simulink model "full_correlator"  (R2022a)
settings: Solver=VariableStepDiscrete  StartTime=0.0  StopTime=4000  RelTol=1e-3
libraries: hdlBasic x2638, hdlSSR x215, hdlDSPIP x4, xbsIndex_r4 x1, xps_library x1
(part 9 of 43)

== system full_correlator/Subsystem2/shared_bram3/sim_mem ==
  addr : Inport
  data : Inport  Port=2
  we : Inport  Port=3
  Data Type Conversion : DataTypeConversion  OutDataTypeStr=single  SaturateOnIntegerOverflow=off  RndMeth=Floor
  Data Type Conversion1 : DataTypeConversion  OutDataTypeStr=double  SaturateOnIntegerOverflow=off  RndMeth=Floor
  Data Type Conversion2 : DataTypeConversion  OutDataTypeStr=boolean  SaturateOnIntegerOverflow=off  RndMeth=Floor
  sfunc : M-S-Function  FunctionName=shared_bram_sim_sfunc  Parameters=depth_bits, latency, init_vals  mask{depth_bits=addr_width, latency=csp_latency, init_vals=init_vals}
      mask prompts: depth_bits "Depth (2^?):"; latency "Latency (>=1):"; init_vals "Initial values:"
      mask Callback latency:
      | latency = str2double(get_param(gcb, 'latency'));
      | if latency < 1
      |     errordlg('Cannot have latency less than one.');
      |     set_param(gcb, 'latency', '1');
      | end
  sim_addr : hdlBasic/Gateway Out  inherit_from_input=off  hdl_port=off  rows=1  columns=1  UseAsDAC=off  DACChannel='1'  interface=None  automatic_assignment=on  address_offset=hex2dec('00')  intf_name=''  intf_description=''  timing_constraint=None  locs_specified=off  LOCs={}  io_standard={}  XmcBlockStatus=1  maskContainerNames=group4  block_type=gatewayout  block_config=sysgen:gateway_out_config  block_width_w=590  block_height_w=620  block_width=620  block_height=750
  sim_data : hdlBasic/Gateway Out  inherit_from_input=off  hdl_port=off  rows=1  columns=1  UseAsDAC=off  DACChannel='1'  interface=None  automatic_assignment=on  address_offset=hex2dec('00')  intf_name=''  intf_description=''  timing_constraint=None  locs_specified=off  LOCs={}  io_standard={}  XmcBlockStatus=1  maskContainerNames=group4  block_type=gatewayout  block_config=sysgen:gateway_out_config  block_width_w=590  block_height_w=620  block_width=620  block_height=750
  sim_we : hdlBasic/Gateway Out  inherit_from_input=off  hdl_port=off  rows=1  columns=1  UseAsDAC=off  DACChannel='1'  interface=None  automatic_assignment=on  address_offset=hex2dec('00')  intf_name=''  intf_description=''  timing_constraint=None  locs_specified=off  LOCs={}  io_standard={}  XmcBlockStatus=1  maskContainerNames=group4  block_type=gatewayout  block_config=sysgen:gateway_out_config  block_width_w=590  block_height_w=620  block_width=620  block_height=750
  data_out : Outport  VectorParamsAs1DForOutWhenUnconnected=off
  wires:
  sfunc/1 -> data_out/1  "output"
  Data Type Conversion2/1 -> sfunc/3  "we"
  Data Type Conversion1/1 -> sfunc/2  "data_in"
  Data Type Conversion/1 -> sfunc/1  "addr"
  sim_we/1 -> Data Type Conversion2/1
  sim_data/1 -> Data Type Conversion1/1
  sim_addr/1 -> Data Type Conversion/1
  we/1 -> sim_we/1
  data/1 -> sim_data/1
  addr/1 -> sim_addr/1

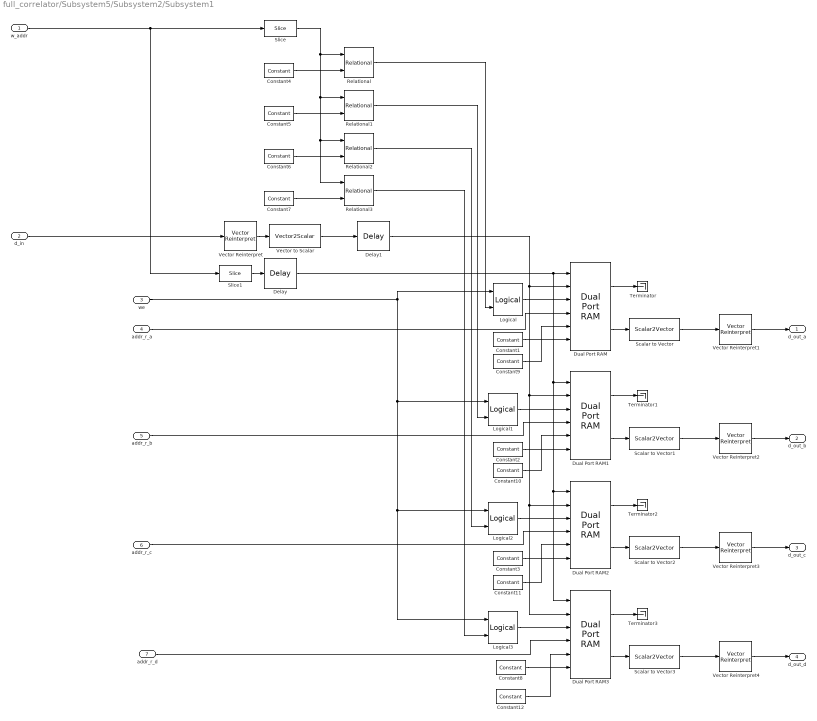
== system full_correlator/Subsystem5/Subsystem2/Subsystem1 ==
  w_addr : Inport
  d_in : Inport  Port=2
  we : Inport  Port=3
  addr_r_a : Inport  Port=4
  addr_r_b : Inport  Port=5
  addr_r_c : Inport  Port=6
  addr_r_d : Inport  Port=7
  Constant{1..3,8} (4 alike) : hdlBasic/Constant  const=0  gui_display_data_type=Boolean  arith_type=Boolean  n_bits=16  bin_pt=14  preci_type=Single  exp_width=8  frac_width=24  explicit_period=on  period=1  XmcBlockStatus=1  maskContainerNames=tabcontainer1  block_type=constant  block_config=sysgen:Constant_config
  Constant{9..12} (4 alike) : hdlBasic/Constant  const=0  gui_display_data_type=Fixed-point  arith_type=Unsigned  n_bits=288  bin_pt=0  preci_type=Single  exp_width=8  frac_width=24  explicit_period=on  period=1  XmcBlockStatus=1  maskContainerNames=tabcontainer1  block_type=constant  block_config=sysgen:Constant_config
  Constant4 : hdlBasic/Constant  const=0  gui_display_data_type=Fixed-point  arith_type=Unsigned  n_bits=2  bin_pt=0  preci_type=Single  exp_width=8  frac_width=24  explicit_period=on  period=1  XmcBlockStatus=1  maskContainerNames=tabcontainer1  block_type=constant  block_config=sysgen:Constant_config
  Constant5 : hdlBasic/Constant  const=1  gui_display_data_type=Fixed-point  arith_type=Unsigned  n_bits=2  bin_pt=0  preci_type=Single  exp_width=8  frac_width=24  explicit_period=on  period=1  XmcBlockStatus=1  maskContainerNames=tabcontainer1  block_type=constant  block_config=sysgen:Constant_config
  Constant6 : hdlBasic/Constant  const=2  gui_display_data_type=Fixed-point  arith_type=Unsigned  n_bits=2  bin_pt=0  preci_type=Single  exp_width=8  frac_width=24  explicit_period=on  period=1  XmcBlockStatus=1  maskContainerNames=tabcontainer1  block_type=constant  block_config=sysgen:Constant_config
  Constant7 : hdlBasic/Constant  const=3  gui_display_data_type=Fixed-point  arith_type=Unsigned  n_bits=2  bin_pt=0  preci_type=Single  exp_width=8  frac_width=24  explicit_period=on  period=1  XmcBlockStatus=1  maskContainerNames=tabcontainer1  block_type=constant  block_config=sysgen:Constant_config
  Delay : hdlBasic/Delay  rst=off  en=off  latency=2  reg_retiming=off  XmcBlockStatus=1  maskContainerNames=group1  block_type=delay  block_config=sysgen:Delay_config
  Delay1 : hdlBasic/Delay  rst=off  en=off  latency=2  reg_retiming=off  XmcBlockStatus=1  maskContainerNames=group1  block_type=delay  block_config=sysgen:Delay_config
  Dual Port RAM{,1..3} (4 alike) : hdlBasic/Dual Port RAM  depth=16  initVector=zeros(1, 16)  distributed_mem=Block RAM  init_a=0  init_b=0  rst_a=off  rst_b=off  en_a=off  en_b=off  latency=1  write_mode_A=Read After Write  write_mode_B=Read After Write  explicit_period=[]  period=[]  simulation_type=fast_sim  XmcBlockStatus=1  maskContainerNames=tabcontainer1  block_type=dpram  block_config=sysgen:Dpram_config  optimize=Area
      settings: infoedit=[]
  Logical{,1..3} (4 alike) : hdlBasic/Logical  logical_function=AND  inputs=2  en=off  latency=1  precision=Full  arith_type=Unsigned  n_bits=16  bin_pt=0  align_bp=on  overflow=[]  quantization=[]  XmcBlockStatus=1  maskContainerNames=tabcontainer1  block_type=logical  block_config=sysgen:Logical_config
  Relational{,1..3} (4 alike) : hdlBasic/Relational  mode=a=b  op_type=Bool  en=off  latency=1  XmcBlockStatus=1  maskContainerNames=tabcontainer1  block_type=relational  block_config=sysgen:Relational_config
  Scalar to Vector{,1..3} (4 alike) : hdlSSR/Scalar2Vector  Width=18  sg_ssr=16  block_type=scalar2vector_ssr  XmcBlockStatus=1  sg_ssr_prev=16  maskContainerNames=group1
  Slice : hdlBasic/Slice  nbits=2  boolean_output=off  mode=Upper Bit Location + Width  bit1=0  base1=MSB of Input  bit0=0  base0=LSB of Input  XmcBlockStatus=1  maskContainerNames=group1  block_type=slice  block_config=sysgen:Slice_config
  Slice1 : hdlBasic/Slice  nbits=4  boolean_output=off  mode=Upper Bit Location + Width  bit1=-2  base1=MSB of Input  bit0=0  base0=LSB of Input  XmcBlockStatus=1  maskContainerNames=group1  block_type=slice  block_config=sysgen:Slice_config
  Terminator{,1..3} (4 alike) : Terminator
  Vector Reinterpret : hdlSSR/Vector Reinterpret  force_arith_type=on  arith_type=Unsigned  force_bin_pt=on  bin_pt=0  sg_ssr=16  block_type=reinterpret_ssr  XmcBlockStatus=1  sg_ssr_prev=16  maskContainerNames=group1
  Vector Reinterpret{1..4} (4 alike) : hdlSSR/Vector Reinterpret  force_arith_type=on  arith_type="Signed  (2's comp)"  force_bin_pt=on  bin_pt=17  sg_ssr=16  block_type=reinterpret_ssr  XmcBlockStatus=1  sg_ssr_prev=16  maskContainerNames=group1
  Vector to Scalar : hdlSSR/Vector2Scalar  sg_ssr=16  block_type=vector2scalar_ssr  XmcBlockStatus=1  sg_ssr_prev=16  maskContainerNames=group1
  d_out_a : Outport
  d_out_b : Outport  Port=2
  d_out_c : Outport  Port=3
  d_out_d : Outport  Port=4
  wires:
  addr_r_b/1 -> Dual Port RAM1/4
  Constant12/1 -> Dual Port RAM3/5
  addr_r_c/1 -> Dual Port RAM2/4
  Relational/1 -> Logical/2
  Constant6/1 -> Relational2/2
  Dual Port RAM1/1 -> Terminator1/1
  Constant11/1 -> Dual Port RAM2/5
  Vector Reinterpret/1 -> Vector to Scalar/1
  Relational3/1 -> Logical3/2
  Constant7/1 -> Relational3/2
  Dual Port RAM/1 -> Terminator/1
  Delay/1 -> Dual Port RAM3/1, Dual Port RAM2/1, Dual Port RAM1/1, Dual Port RAM/1
  Vector to Scalar/1 -> Delay1/1
  Logical2/1 -> Dual Port RAM2/3
  d_in/1 -> Vector Reinterpret/1
  Constant3/1 -> Dual Port RAM2/6
  Dual Port RAM1/2 -> Scalar to Vector1/1
  Delay1/1 -> Dual Port RAM3/2, Dual Port RAM2/2, Dual Port RAM1/2, Dual Port RAM/2
  Relational1/1 -> Logical1/2
  we/1 -> Logical3/1, Logical2/1, Logical1/1, Logical/1
  Slice/1 -> Relational3/1, Relational2/1, Relational1/1, Relational/1
  Constant9/1 -> Dual Port RAM/5
  Constant1/1 -> Dual Port RAM/6
  Dual Port RAM2/1 -> Terminator2/1
  Constant10/1 -> Dual Port RAM1/5
  w_addr/1 -> Slice1/1, Slice/1
  Dual Port RAM3/2 -> Scalar to Vector3/1
  Logical/1 -> Dual Port RAM/3
  Constant2/1 -> Dual Port RAM1/6
  Constant8/1 -> Dual Port RAM3/6
  Constant4/1 -> Relational/2
  Dual Port RAM3/1 -> Terminator3/1
  Logical1/1 -> Dual Port RAM1/3
  Logical3/1 -> Dual Port RAM3/3
  Constant5/1 -> Relational1/2
  Dual Port RAM2/2 -> Scalar to Vector2/1
  addr_r_d/1 -> Dual Port RAM3/4
  Slice1/1 -> Delay/1
  Relational2/1 -> Logical2/2
  addr_r_a/1 -> Dual Port RAM/4
  Dual Port RAM/2 -> Scalar to Vector/1
  Scalar to Vector/1 -> Vector Reinterpret1/1
  Scalar to Vector1/1 -> Vector Reinterpret2/1
  Scalar to Vector2/1 -> Vector Reinterpret3/1
  Scalar to Vector3/1 -> Vector Reinterpret4/1
  Vector Reinterpret1/1 -> d_out_a/1
  Vector Reinterpret2/1 -> d_out_b/1
  Vector Reinterpret3/1 -> d_out_c/1
  Vector Reinterpret4/1 -> d_out_d/1

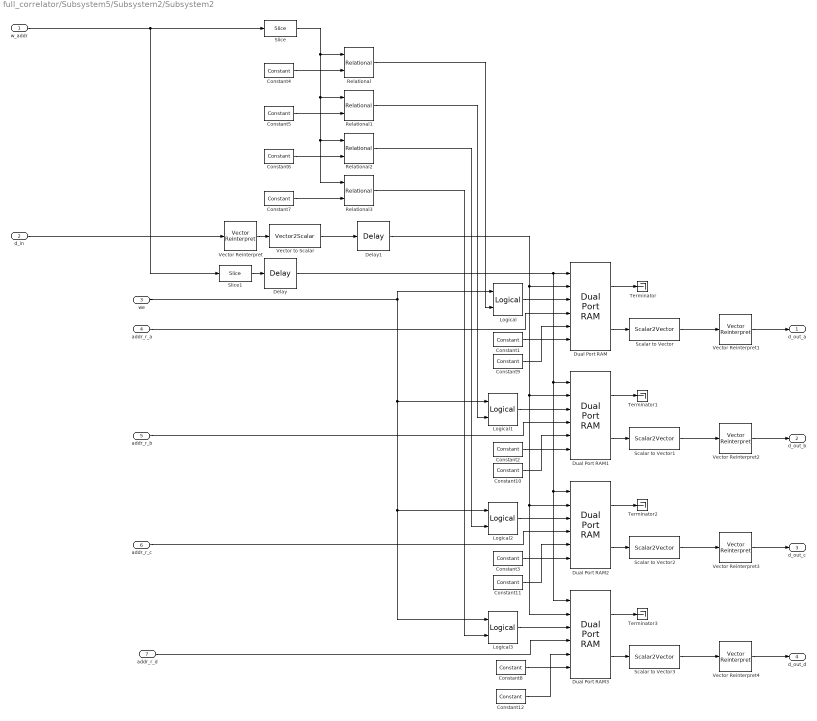
== system full_correlator/Subsystem5/Subsystem2/Subsystem2 ==
  w_addr : Inport
  d_in : Inport  Port=2
  we : Inport  Port=3
  addr_r_a : Inport  Port=4
  addr_r_b : Inport  Port=5
  addr_r_c : Inport  Port=6
  addr_r_d : Inport  Port=7
  Constant{1..3,8} (4 alike) : hdlBasic/Constant  const=0  gui_display_data_type=Boolean  arith_type=Boolean  n_bits=16  bin_pt=14  preci_type=Single  exp_width=8  frac_width=24  explicit_period=on  period=1  XmcBlockStatus=1  maskContainerNames=tabcontainer1  block_type=constant  block_config=sysgen:Constant_config
  Constant{9..12} (4 alike) : hdlBasic/Constant  const=0  gui_display_data_type=Fixed-point  arith_type=Unsigned  n_bits=288  bin_pt=0  preci_type=Single  exp_width=8  frac_width=24  explicit_period=on  period=1  XmcBlockStatus=1  maskContainerNames=tabcontainer1  block_type=constant  block_config=sysgen:Constant_config
  Constant4 : hdlBasic/Constant  const=0  gui_display_data_type=Fixed-point  arith_type=Unsigned  n_bits=2  bin_pt=0  preci_type=Single  exp_width=8  frac_width=24  explicit_period=on  period=1  XmcBlockStatus=1  maskContainerNames=tabcontainer1  block_type=constant  block_config=sysgen:Constant_config
  Constant5 : hdlBasic/Constant  const=1  gui_display_data_type=Fixed-point  arith_type=Unsigned  n_bits=2  bin_pt=0  preci_type=Single  exp_width=8  frac_width=24  explicit_period=on  period=1  XmcBlockStatus=1  maskContainerNames=tabcontainer1  block_type=constant  block_config=sysgen:Constant_config
  Constant6 : hdlBasic/Constant  const=2  gui_display_data_type=Fixed-point  arith_type=Unsigned  n_bits=2  bin_pt=0  preci_type=Single  exp_width=8  frac_width=24  explicit_period=on  period=1  XmcBlockStatus=1  maskContainerNames=tabcontainer1  block_type=constant  block_config=sysgen:Constant_config
  Constant7 : hdlBasic/Constant  const=3  gui_display_data_type=Fixed-point  arith_type=Unsigned  n_bits=2  bin_pt=0  preci_type=Single  exp_width=8  frac_width=24  explicit_period=on  period=1  XmcBlockStatus=1  maskContainerNames=tabcontainer1  block_type=constant  block_config=sysgen:Constant_config
  Delay : hdlBasic/Delay  rst=off  en=off  latency=2  reg_retiming=off  XmcBlockStatus=1  maskContainerNames=group1  block_type=delay  block_config=sysgen:Delay_config
  Delay1 : hdlBasic/Delay  rst=off  en=off  latency=2  reg_retiming=off  XmcBlockStatus=1  maskContainerNames=group1  block_type=delay  block_config=sysgen:Delay_config
  Dual Port RAM{,1..3} (4 alike) : hdlBasic/Dual Port RAM  depth=16  initVector=zeros(1, 16)  distributed_mem=Block RAM  init_a=0  init_b=0  rst_a=off  rst_b=off  en_a=off  en_b=off  latency=1  write_mode_A=Read After Write  write_mode_B=Read After Write  explicit_period=[]  period=[]  simulation_type=fast_sim  XmcBlockStatus=1  maskContainerNames=tabcontainer1  block_type=dpram  block_config=sysgen:Dpram_config  optimize=Area
      settings: infoedit=[]
  Logical{,1..3} (4 alike) : hdlBasic/Logical  logical_function=AND  inputs=2  en=off  latency=1  precision=Full  arith_type=Unsigned  n_bits=16  bin_pt=0  align_bp=on  overflow=[]  quantization=[]  XmcBlockStatus=1  maskContainerNames=tabcontainer1  block_type=logical  block_config=sysgen:Logical_config
  Relational{,1..3} (4 alike) : hdlBasic/Relational  mode=a=b  op_type=Bool  en=off  latency=1  XmcBlockStatus=1  maskContainerNames=tabcontainer1  block_type=relational  block_config=sysgen:Relational_config
  Scalar to Vector{,1..3} (4 alike) : hdlSSR/Scalar2Vector  Width=18  sg_ssr=16  block_type=scalar2vector_ssr  XmcBlockStatus=1  sg_ssr_prev=16  maskContainerNames=group1
  Slice : hdlBasic/Slice  nbits=2  boolean_output=off  mode=Upper Bit Location + Width  bit1=0  base1=MSB of Input  bit0=0  base0=LSB of Input  XmcBlockStatus=1  maskContainerNames=group1  block_type=slice  block_config=sysgen:Slice_config
  Slice1 : hdlBasic/Slice  nbits=4  boolean_output=off  mode=Upper Bit Location + Width  bit1=-2  base1=MSB of Input  bit0=0  base0=LSB of Input  XmcBlockStatus=1  maskContainerNames=group1  block_type=slice  block_config=sysgen:Slice_config
  Terminator{,1..3} (4 alike) : Terminator
  Vector Reinterpret : hdlSSR/Vector Reinterpret  force_arith_type=on  arith_type=Unsigned  force_bin_pt=on  bin_pt=0  sg_ssr=16  block_type=reinterpret_ssr  XmcBlockStatus=1  sg_ssr_prev=16  maskContainerNames=group1
  Vector Reinterpret{1..4} (4 alike) : hdlSSR/Vector Reinterpret  force_arith_type=on  arith_type="Signed  (2's comp)"  force_bin_pt=on  bin_pt=17  sg_ssr=16  block_type=reinterpret_ssr  XmcBlockStatus=1  sg_ssr_prev=16  maskContainerNames=group1
  Vector to Scalar : hdlSSR/Vector2Scalar  sg_ssr=16  block_type=vector2scalar_ssr  XmcBlockStatus=1  sg_ssr_prev=16  maskContainerNames=group1
  d_out_a : Outport
  d_out_b : Outport  Port=2
  d_out_c : Outport  Port=3
  d_out_d : Outport  Port=4
  wires:
  addr_r_b/1 -> Dual Port RAM1/4
  Constant12/1 -> Dual Port RAM3/5
  addr_r_c/1 -> Dual Port RAM2/4
  Relational/1 -> Logical/2
  Constant6/1 -> Relational2/2
  Dual Port RAM1/1 -> Terminator1/1
  Constant11/1 -> Dual Port RAM2/5
  Vector Reinterpret/1 -> Vector to Scalar/1
  Relational3/1 -> Logical3/2
  Constant7/1 -> Relational3/2
  Dual Port RAM/1 -> Terminator/1
  Delay/1 -> Dual Port RAM3/1, Dual Port RAM2/1, Dual Port RAM1/1, Dual Port RAM/1
  Vector to Scalar/1 -> Delay1/1
  Logical2/1 -> Dual Port RAM2/3
  d_in/1 -> Vector Reinterpret/1
  Constant3/1 -> Dual Port RAM2/6
  Dual Port RAM1/2 -> Scalar to Vector1/1
  Delay1/1 -> Dual Port RAM3/2, Dual Port RAM2/2, Dual Port RAM1/2, Dual Port RAM/2
  Relational1/1 -> Logical1/2
  we/1 -> Logical3/1, Logical2/1, Logical1/1, Logical/1
  Slice/1 -> Relational3/1, Relational2/1, Relational1/1, Relational/1
  Constant9/1 -> Dual Port RAM/5
  Constant1/1 -> Dual Port RAM/6
  Dual Port RAM2/1 -> Terminator2/1
  Constant10/1 -> Dual Port RAM1/5
  w_addr/1 -> Slice1/1, Slice/1
  Dual Port RAM3/2 -> Scalar to Vector3/1
  Logical/1 -> Dual Port RAM/3
  Constant2/1 -> Dual Port RAM1/6
  Constant8/1 -> Dual Port RAM3/6
  Constant4/1 -> Relational/2
  Dual Port RAM3/1 -> Terminator3/1
  Logical1/1 -> Dual Port RAM1/3
  Logical3/1 -> Dual Port RAM3/3
  Constant5/1 -> Relational1/2
  Dual Port RAM2/2 -> Scalar to Vector2/1
  addr_r_d/1 -> Dual Port RAM3/4
  Slice1/1 -> Delay/1
  Relational2/1 -> Logical2/2
  addr_r_a/1 -> Dual Port RAM/4
  Dual Port RAM/2 -> Scalar to Vector/1
  Scalar to Vector/1 -> Vector Reinterpret1/1
  Scalar to Vector1/1 -> Vector Reinterpret2/1
  Scalar to Vector2/1 -> Vector Reinterpret3/1
  Scalar to Vector3/1 -> Vector Reinterpret4/1
  Vector Reinterpret1/1 -> d_out_a/1
  Vector Reinterpret2/1 -> d_out_b/1
  Vector Reinterpret3/1 -> d_out_c/1
  Vector Reinterpret4/1 -> d_out_d/1

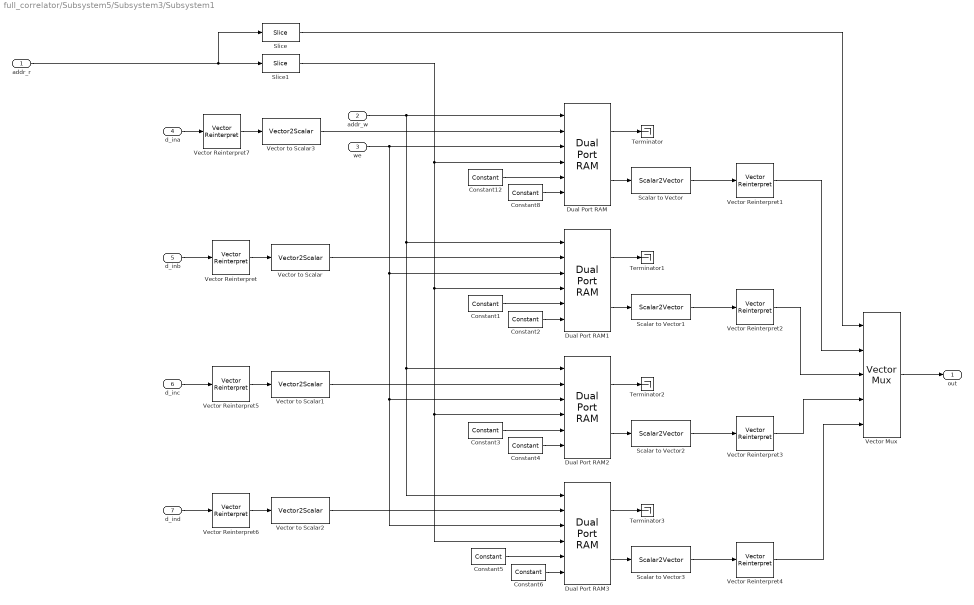
== system full_correlator/Subsystem5/Subsystem3/Subsystem1 ==
  addr_r : Inport
  addr_w : Inport  Port=2
  we : Inport  Port=3
  d_ina : Inport  Port=4
  d_inb : Inport  Port=5
  d_inc : Inport  Port=6
  d_ind : Inport  Port=7
  Constant{1,3,5,12} (4 alike) : hdlBasic/Constant  const=0  gui_display_data_type=Fixed-point  arith_type=Unsigned  n_bits=288  bin_pt=0  preci_type=Single  exp_width=8  frac_width=24  explicit_period=on  period=1  XmcBlockStatus=1  maskContainerNames=tabcontainer1  block_type=constant  block_config=sysgen:Constant_config
  Constant{2,4,6,8} (4 alike) : hdlBasic/Constant  const=0  gui_display_data_type=Boolean  arith_type=Boolean  n_bits=16  bin_pt=14  preci_type=Single  exp_width=8  frac_width=24  explicit_period=on  period=1  XmcBlockStatus=1  maskContainerNames=tabcontainer1  block_type=constant  block_config=sysgen:Constant_config
  Dual Port RAM{,1..3} (4 alike) : hdlBasic/Dual Port RAM  depth=16  initVector=zeros(1, 16)  distributed_mem=Block RAM  init_a=0  init_b=0  rst_a=off  rst_b=off  en_a=off  en_b=off  latency=1  write_mode_A=Read After Write  write_mode_B=Read After Write  explicit_period=[]  period=[]  simulation_type=fast_sim  XmcBlockStatus=1  maskContainerNames=tabcontainer1  block_type=dpram  block_config=sysgen:Dpram_config  optimize=Area
      settings: infoedit=[]
  Scalar to Vector{,1..3} (4 alike) : hdlSSR/Scalar2Vector  Width=18  sg_ssr=16  block_type=scalar2vector_ssr  XmcBlockStatus=1  sg_ssr_prev=16  maskContainerNames=group1
  Slice : hdlBasic/Slice  nbits=2  boolean_output=off  mode=Upper Bit Location + Width  bit1=0  base1=MSB of Input  bit0=0  base0=LSB of Input  XmcBlockStatus=1  maskContainerNames=group1  block_type=slice  block_config=sysgen:Slice_config
  Slice1 : hdlBasic/Slice  nbits=4  boolean_output=off  mode=Upper Bit Location + Width  bit1=-2  base1=MSB of Input  bit0=0  base0=LSB of Input  XmcBlockStatus=1  maskContainerNames=group1  block_type=slice  block_config=sysgen:Slice_config
  Terminator{,1..3} (4 alike) : Terminator
  Vector Mux : hdlSSR/Vector Mux  inputs=4  en=off  vectorize_en=off  vectorize_sel=off  sg_latency=1  sg_ssr=16  precision=Full  arith_type=Unsigned  n_bits=16  bin_pt=14  quantization=Truncate  overflow=Wrap  block_type=mux_ssr  inputs_prev=2  XmcBlockStatus=1  sg_ssr_prev=16  maskContainerNames=group1
  Vector Reinterpret{,5..7} (4 alike) : hdlSSR/Vector Reinterpret  force_arith_type=on  arith_type=Unsigned  force_bin_pt=on  bin_pt=0  sg_ssr=16  block_type=reinterpret_ssr  XmcBlockStatus=1  sg_ssr_prev=16  maskContainerNames=group1
  Vector Reinterpret{1..4} (4 alike) : hdlSSR/Vector Reinterpret  force_arith_type=on  arith_type="Signed  (2's comp)"  force_bin_pt=on  bin_pt=17  sg_ssr=16  block_type=reinterpret_ssr  XmcBlockStatus=1  sg_ssr_prev=16  maskContainerNames=group1
  Vector to Scalar{,1..3} (4 alike) : hdlSSR/Vector2Scalar  sg_ssr=16  block_type=vector2scalar_ssr  XmcBlockStatus=1  sg_ssr_prev=16  maskContainerNames=group1
  out : Outport
  wires:
  Dual Port RAM1/1 -> Terminator1/1
  Dual Port RAM/1 -> Terminator/1
  Dual Port RAM1/2 -> Scalar to Vector1/1
  Dual Port RAM2/1 -> Terminator2/1
  Dual Port RAM3/2 -> Scalar to Vector3/1
  Dual Port RAM3/1 -> Terminator3/1
  Dual Port RAM2/2 -> Scalar to Vector2/1
  Dual Port RAM/2 -> Scalar to Vector/1
  Scalar to Vector/1 -> Vector Reinterpret1/1
  Scalar to Vector1/1 -> Vector Reinterpret2/1
  Scalar to Vector2/1 -> Vector Reinterpret3/1
  Scalar to Vector3/1 -> Vector Reinterpret4/1
  addr_w/1 -> Dual Port RAM3/1, Dual Port RAM2/1, Dual Port RAM1/1, Dual Port RAM/1
  Vector to Scalar3/1 -> Dual Port RAM/2
  Vector to Scalar/1 -> Dual Port RAM1/2
  Vector to Scalar1/1 -> Dual Port RAM2/2
  Vector to Scalar2/1 -> Dual Port RAM3/2
  we/1 -> Dual Port RAM3/3, Dual Port RAM2/3, Dual Port RAM1/3, Dual Port RAM/3
  Vector Reinterpret/1 -> Vector to Scalar/1
  Vector Reinterpret5/1 -> Vector to Scalar1/1
  Vector Reinterpret6/1 -> Vector to Scalar2/1
  Vector Reinterpret7/1 -> Vector to Scalar3/1
  Vector Mux/1 -> out/1
  Vector Reinterpret1/1 -> Vector Mux/2
  Vector Reinterpret2/1 -> Vector Mux/3
  Vector Reinterpret3/1 -> Vector Mux/4
  Vector Reinterpret4/1 -> Vector Mux/5
  Constant8/1 -> Dual Port RAM/6
  Constant12/1 -> Dual Port RAM/5
  Constant2/1 -> Dual Port RAM1/6
  Constant1/1 -> Dual Port RAM1/5
  Constant4/1 -> Dual Port RAM2/6
  Constant3/1 -> Dual Port RAM2/5
  Constant6/1 -> Dual Port RAM3/6
  Constant5/1 -> Dual Port RAM3/5
  addr_r/1 -> Slice/1, Slice1/1
  Slice/1 -> Vector Mux/1
  Slice1/1 -> Dual Port RAM3/4, Dual Port RAM2/4, Dual Port RAM1/4, Dual Port RAM/4
  d_ina/1 -> Vector Reinterpret7/1
  d_inb/1 -> Vector Reinterpret/1
  d_inc/1 -> Vector Reinterpret5/1
  d_ind/1 -> Vector Reinterpret6/1

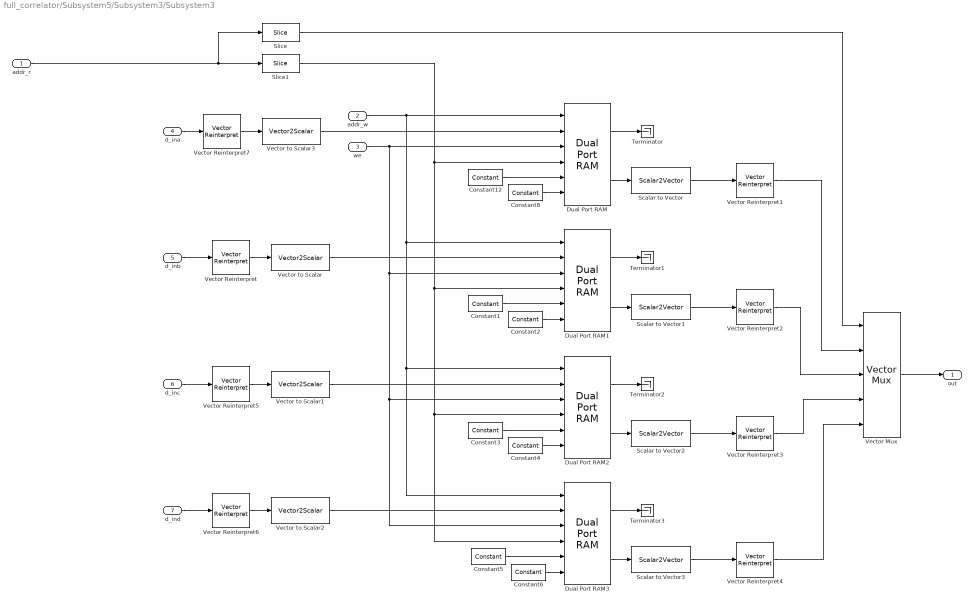
== system full_correlator/Subsystem5/Subsystem3/Subsystem3 ==
  addr_r : Inport
  addr_w : Inport  Port=2
  we : Inport  Port=3
  d_ina : Inport  Port=4
  d_inb : Inport  Port=5
  d_inc : Inport  Port=6
  d_ind : Inport  Port=7
  Constant{1,3,5,12} (4 alike) : hdlBasic/Constant  const=0  gui_display_data_type=Fixed-point  arith_type=Unsigned  n_bits=288  bin_pt=0  preci_type=Single  exp_width=8  frac_width=24  explicit_period=on  period=1  XmcBlockStatus=1  maskContainerNames=tabcontainer1  block_type=constant  block_config=sysgen:Constant_config
  Constant{2,4,6,8} (4 alike) : hdlBasic/Constant  const=0  gui_display_data_type=Boolean  arith_type=Boolean  n_bits=16  bin_pt=14  preci_type=Single  exp_width=8  frac_width=24  explicit_period=on  period=1  XmcBlockStatus=1  maskContainerNames=tabcontainer1  block_type=constant  block_config=sysgen:Constant_config
  Dual Port RAM{,1..3} (4 alike) : hdlBasic/Dual Port RAM  depth=16  initVector=zeros(1, 16)  distributed_mem=Block RAM  init_a=0  init_b=0  rst_a=off  rst_b=off  en_a=off  en_b=off  latency=1  write_mode_A=Read After Write  write_mode_B=Read After Write  explicit_period=[]  period=[]  simulation_type=fast_sim  XmcBlockStatus=1  maskContainerNames=tabcontainer1  block_type=dpram  block_config=sysgen:Dpram_config  optimize=Area
      settings: infoedit=[]
  Scalar to Vector{,1..3} (4 alike) : hdlSSR/Scalar2Vector  Width=18  sg_ssr=16  block_type=scalar2vector_ssr  XmcBlockStatus=1  sg_ssr_prev=16  maskContainerNames=group1
  Slice : hdlBasic/Slice  nbits=2  boolean_output=off  mode=Upper Bit Location + Width  bit1=0  base1=MSB of Input  bit0=0  base0=LSB of Input  XmcBlockStatus=1  maskContainerNames=group1  block_type=slice  block_config=sysgen:Slice_config
  Slice1 : hdlBasic/Slice  nbits=4  boolean_output=off  mode=Upper Bit Location + Width  bit1=-2  base1=MSB of Input  bit0=0  base0=LSB of Input  XmcBlockStatus=1  maskContainerNames=group1  block_type=slice  block_config=sysgen:Slice_config
  Terminator{,1..3} (4 alike) : Terminator
  Vector Mux : hdlSSR/Vector Mux  inputs=4  en=off  vectorize_en=off  vectorize_sel=off  sg_latency=1  sg_ssr=16  precision=Full  arith_type=Unsigned  n_bits=16  bin_pt=14  quantization=Truncate  overflow=Wrap  block_type=mux_ssr  inputs_prev=2  XmcBlockStatus=1  sg_ssr_prev=16  maskContainerNames=group1
  Vector Reinterpret{,5..7} (4 alike) : hdlSSR/Vector Reinterpret  force_arith_type=on  arith_type=Unsigned  force_bin_pt=on  bin_pt=0  sg_ssr=16  block_type=reinterpret_ssr  XmcBlockStatus=1  sg_ssr_prev=16  maskContainerNames=group1
  Vector Reinterpret{1..4} (4 alike) : hdlSSR/Vector Reinterpret  force_arith_type=on  arith_type="Signed  (2's comp)"  force_bin_pt=on  bin_pt=17  sg_ssr=16  block_type=reinterpret_ssr  XmcBlockStatus=1  sg_ssr_prev=16  maskContainerNames=group1
  Vector to Scalar{,1..3} (4 alike) : hdlSSR/Vector2Scalar  sg_ssr=16  block_type=vector2scalar_ssr  XmcBlockStatus=1  sg_ssr_prev=16  maskContainerNames=group1
  out : Outport
  wires:
  Dual Port RAM1/1 -> Terminator1/1
  Dual Port RAM/1 -> Terminator/1
  Dual Port RAM1/2 -> Scalar to Vector1/1
  Dual Port RAM2/1 -> Terminator2/1
  Dual Port RAM3/2 -> Scalar to Vector3/1
  Dual Port RAM3/1 -> Terminator3/1
  Dual Port RAM2/2 -> Scalar to Vector2/1
  Dual Port RAM/2 -> Scalar to Vector/1
  Scalar to Vector/1 -> Vector Reinterpret1/1
  Scalar to Vector1/1 -> Vector Reinterpret2/1
  Scalar to Vector2/1 -> Vector Reinterpret3/1
  Scalar to Vector3/1 -> Vector Reinterpret4/1
  addr_w/1 -> Dual Port RAM3/1, Dual Port RAM2/1, Dual Port RAM1/1, Dual Port RAM/1
  Vector to Scalar3/1 -> Dual Port RAM/2
  Vector to Scalar/1 -> Dual Port RAM1/2
  Vector to Scalar1/1 -> Dual Port RAM2/2
  Vector to Scalar2/1 -> Dual Port RAM3/2
  we/1 -> Dual Port RAM3/3, Dual Port RAM2/3, Dual Port RAM1/3, Dual Port RAM/3
  Vector Reinterpret/1 -> Vector to Scalar/1
  Vector Reinterpret5/1 -> Vector to Scalar1/1
  Vector Reinterpret6/1 -> Vector to Scalar2/1
  Vector Reinterpret7/1 -> Vector to Scalar3/1
  Vector Mux/1 -> out/1
  Vector Reinterpret1/1 -> Vector Mux/2
  Vector Reinterpret2/1 -> Vector Mux/3
  Vector Reinterpret3/1 -> Vector Mux/4
  Vector Reinterpret4/1 -> Vector Mux/5
  Constant8/1 -> Dual Port RAM/6
  Constant12/1 -> Dual Port RAM/5
  Constant2/1 -> Dual Port RAM1/6
  Constant1/1 -> Dual Port RAM1/5
  Constant4/1 -> Dual Port RAM2/6
  Constant3/1 -> Dual Port RAM2/5
  Constant6/1 -> Dual Port RAM3/6
  Constant5/1 -> Dual Port RAM3/5
  addr_r/1 -> Slice/1, Slice1/1
  Slice/1 -> Vector Mux/1
  Slice1/1 -> Dual Port RAM3/4, Dual Port RAM2/4, Dual Port RAM1/4, Dual Port RAM/4
  d_ina/1 -> Vector Reinterpret7/1
  d_inb/1 -> Vector Reinterpret/1
  d_inc/1 -> Vector Reinterpret5/1
  d_ind/1 -> Vector Reinterpret6/1

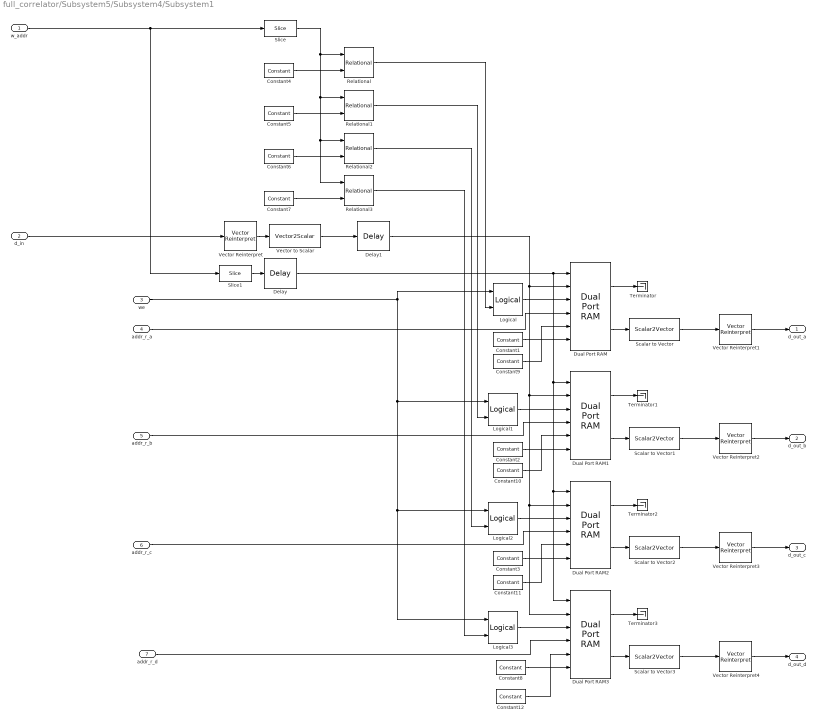
== system full_correlator/Subsystem5/Subsystem4/Subsystem1 ==
  w_addr : Inport
  d_in : Inport  Port=2
  we : Inport  Port=3
  addr_r_a : Inport  Port=4
  addr_r_b : Inport  Port=5
  addr_r_c : Inport  Port=6
  addr_r_d : Inport  Port=7
  Constant{1..3,8} (4 alike) : hdlBasic/Constant  const=0  gui_display_data_type=Boolean  arith_type=Boolean  n_bits=16  bin_pt=14  preci_type=Single  exp_width=8  frac_width=24  explicit_period=on  period=1  XmcBlockStatus=1  maskContainerNames=tabcontainer1  block_type=constant  block_config=sysgen:Constant_config
  Constant{9..12} (4 alike) : hdlBasic/Constant  const=0  gui_display_data_type=Fixed-point  arith_type=Unsigned  n_bits=288  bin_pt=0  preci_type=Single  exp_width=8  frac_width=24  explicit_period=on  period=1  XmcBlockStatus=1  maskContainerNames=tabcontainer1  block_type=constant  block_config=sysgen:Constant_config
  Constant4 : hdlBasic/Constant  const=0  gui_display_data_type=Fixed-point  arith_type=Unsigned  n_bits=2  bin_pt=0  preci_type=Single  exp_width=8  frac_width=24  explicit_period=on  period=1  XmcBlockStatus=1  maskContainerNames=tabcontainer1  block_type=constant  block_config=sysgen:Constant_config
  Constant5 : hdlBasic/Constant  const=1  gui_display_data_type=Fixed-point  arith_type=Unsigned  n_bits=2  bin_pt=0  preci_type=Single  exp_width=8  frac_width=24  explicit_period=on  period=1  XmcBlockStatus=1  maskContainerNames=tabcontainer1  block_type=constant  block_config=sysgen:Constant_config
  Constant6 : hdlBasic/Constant  const=2  gui_display_data_type=Fixed-point  arith_type=Unsigned  n_bits=2  bin_pt=0  preci_type=Single  exp_width=8  frac_width=24  explicit_period=on  period=1  XmcBlockStatus=1  maskContainerNames=tabcontainer1  block_type=constant  block_config=sysgen:Constant_config
  Constant7 : hdlBasic/Constant  const=3  gui_display_data_type=Fixed-point  arith_type=Unsigned  n_bits=2  bin_pt=0  preci_type=Single  exp_width=8  frac_width=24  explicit_period=on  period=1  XmcBlockStatus=1  maskContainerNames=tabcontainer1  block_type=constant  block_config=sysgen:Constant_config
  Delay : hdlBasic/Delay  rst=off  en=off  latency=2  reg_retiming=off  XmcBlockStatus=1  maskContainerNames=group1  block_type=delay  block_config=sysgen:Delay_config
  Delay1 : hdlBasic/Delay  rst=off  en=off  latency=2  reg_retiming=off  XmcBlockStatus=1  maskContainerNames=group1  block_type=delay  block_config=sysgen:Delay_config
  Dual Port RAM{,1..3} (4 alike) : hdlBasic/Dual Port RAM  depth=16  initVector=zeros(1, 16)  distributed_mem=Block RAM  init_a=0  init_b=0  rst_a=off  rst_b=off  en_a=off  en_b=off  latency=1  write_mode_A=Read After Write  write_mode_B=Read After Write  explicit_period=[]  period=[]  simulation_type=fast_sim  XmcBlockStatus=1  maskContainerNames=tabcontainer1  block_type=dpram  block_config=sysgen:Dpram_config  optimize=Area
      settings: infoedit=[]
  Logical{,1..3} (4 alike) : hdlBasic/Logical  logical_function=AND  inputs=2  en=off  latency=1  precision=Full  arith_type=Unsigned  n_bits=16  bin_pt=0  align_bp=on  overflow=[]  quantization=[]  XmcBlockStatus=1  maskContainerNames=tabcontainer1  block_type=logical  block_config=sysgen:Logical_config
  Relational{,1..3} (4 alike) : hdlBasic/Relational  mode=a=b  op_type=Bool  en=off  latency=1  XmcBlockStatus=1  maskContainerNames=tabcontainer1  block_type=relational  block_config=sysgen:Relational_config
  Scalar to Vector{,1..3} (4 alike) : hdlSSR/Scalar2Vector  Width=18  sg_ssr=16  block_type=scalar2vector_ssr  XmcBlockStatus=1  sg_ssr_prev=16  maskContainerNames=group1
  Slice : hdlBasic/Slice  nbits=2  boolean_output=off  mode=Upper Bit Location + Width  bit1=0  base1=MSB of Input  bit0=0  base0=LSB of Input  XmcBlockStatus=1  maskContainerNames=group1  block_type=slice  block_config=sysgen:Slice_config
  Slice1 : hdlBasic/Slice  nbits=4  boolean_output=off  mode=Upper Bit Location + Width  bit1=-2  base1=MSB of Input  bit0=0  base0=LSB of Input  XmcBlockStatus=1  maskContainerNames=group1  block_type=slice  block_config=sysgen:Slice_config
  Terminator{,1..3} (4 alike) : Terminator
  Vector Reinterpret : hdlSSR/Vector Reinterpret  force_arith_type=on  arith_type=Unsigned  force_bin_pt=on  bin_pt=0  sg_ssr=16  block_type=reinterpret_ssr  XmcBlockStatus=1  sg_ssr_prev=16  maskContainerNames=group1
  Vector Reinterpret{1..4} (4 alike) : hdlSSR/Vector Reinterpret  force_arith_type=on  arith_type="Signed  (2's comp)"  force_bin_pt=on  bin_pt=17  sg_ssr=16  block_type=reinterpret_ssr  XmcBlockStatus=1  sg_ssr_prev=16  maskContainerNames=group1
  Vector to Scalar : hdlSSR/Vector2Scalar  sg_ssr=16  block_type=vector2scalar_ssr  XmcBlockStatus=1  sg_ssr_prev=16  maskContainerNames=group1
  d_out_a : Outport
  d_out_b : Outport  Port=2
  d_out_c : Outport  Port=3
  d_out_d : Outport  Port=4
  wires:
  addr_r_b/1 -> Dual Port RAM1/4
  Constant12/1 -> Dual Port RAM3/5
  addr_r_c/1 -> Dual Port RAM2/4
  Relational/1 -> Logical/2
  Constant6/1 -> Relational2/2
  Dual Port RAM1/1 -> Terminator1/1
  Constant11/1 -> Dual Port RAM2/5
  Vector Reinterpret/1 -> Vector to Scalar/1
  Relational3/1 -> Logical3/2
  Constant7/1 -> Relational3/2
  Dual Port RAM/1 -> Terminator/1
  Delay/1 -> Dual Port RAM3/1, Dual Port RAM2/1, Dual Port RAM1/1, Dual Port RAM/1
  Vector to Scalar/1 -> Delay1/1
  Logical2/1 -> Dual Port RAM2/3
  d_in/1 -> Vector Reinterpret/1
  Constant3/1 -> Dual Port RAM2/6
  Dual Port RAM1/2 -> Scalar to Vector1/1
  Delay1/1 -> Dual Port RAM3/2, Dual Port RAM2/2, Dual Port RAM1/2, Dual Port RAM/2
  Relational1/1 -> Logical1/2
  we/1 -> Logical3/1, Logical2/1, Logical1/1, Logical/1
  Slice/1 -> Relational3/1, Relational2/1, Relational1/1, Relational/1
  Constant9/1 -> Dual Port RAM/5
  Constant1/1 -> Dual Port RAM/6
  Dual Port RAM2/1 -> Terminator2/1
  Constant10/1 -> Dual Port RAM1/5
  w_addr/1 -> Slice1/1, Slice/1
  Dual Port RAM3/2 -> Scalar to Vector3/1
  Logical/1 -> Dual Port RAM/3
  Constant2/1 -> Dual Port RAM1/6
  Constant8/1 -> Dual Port RAM3/6
  Constant4/1 -> Relational/2
  Dual Port RAM3/1 -> Terminator3/1
  Logical1/1 -> Dual Port RAM1/3
  Logical3/1 -> Dual Port RAM3/3
  Constant5/1 -> Relational1/2
  Dual Port RAM2/2 -> Scalar to Vector2/1
  addr_r_d/1 -> Dual Port RAM3/4
  Slice1/1 -> Delay/1
  Relational2/1 -> Logical2/2
  addr_r_a/1 -> Dual Port RAM/4
  Dual Port RAM/2 -> Scalar to Vector/1
  Scalar to Vector/1 -> Vector Reinterpret1/1
  Scalar to Vector1/1 -> Vector Reinterpret2/1
  Scalar to Vector2/1 -> Vector Reinterpret3/1
  Scalar to Vector3/1 -> Vector Reinterpret4/1
  Vector Reinterpret1/1 -> d_out_a/1
  Vector Reinterpret2/1 -> d_out_b/1
  Vector Reinterpret3/1 -> d_out_c/1
  Vector Reinterpret4/1 -> d_out_d/1

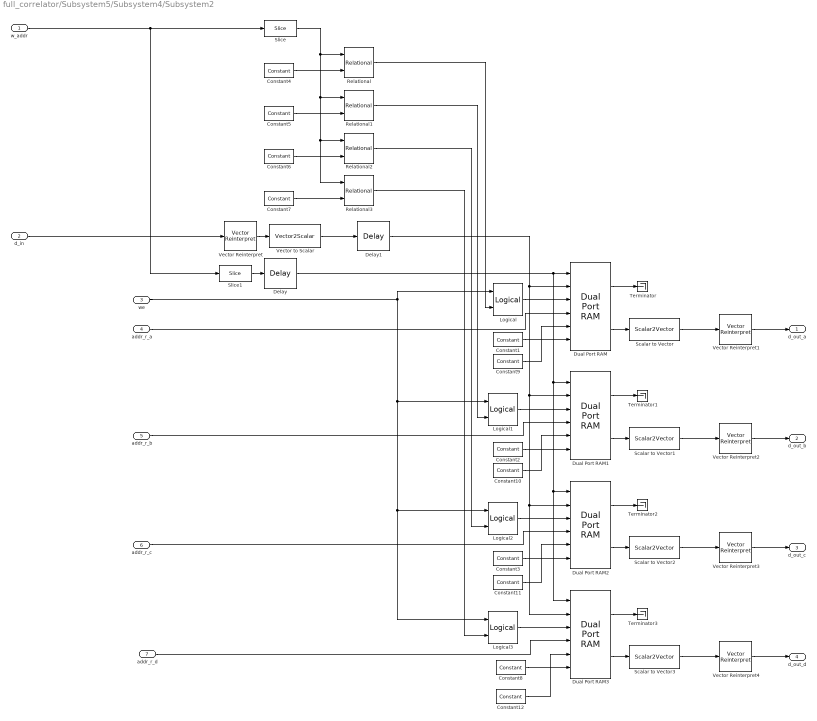
== system full_correlator/Subsystem5/Subsystem4/Subsystem2 ==
  w_addr : Inport
  d_in : Inport  Port=2
  we : Inport  Port=3
  addr_r_a : Inport  Port=4
  addr_r_b : Inport  Port=5
  addr_r_c : Inport  Port=6
  addr_r_d : Inport  Port=7
  Constant{1..3,8} (4 alike) : hdlBasic/Constant  const=0  gui_display_data_type=Boolean  arith_type=Boolean  n_bits=16  bin_pt=14  preci_type=Single  exp_width=8  frac_width=24  explicit_period=on  period=1  XmcBlockStatus=1  maskContainerNames=tabcontainer1  block_type=constant  block_config=sysgen:Constant_config
  Constant{9..12} (4 alike) : hdlBasic/Constant  const=0  gui_display_data_type=Fixed-point  arith_type=Unsigned  n_bits=288  bin_pt=0  preci_type=Single  exp_width=8  frac_width=24  explicit_period=on  period=1  XmcBlockStatus=1  maskContainerNames=tabcontainer1  block_type=constant  block_config=sysgen:Constant_config
  Constant4 : hdlBasic/Constant  const=0  gui_display_data_type=Fixed-point  arith_type=Unsigned  n_bits=2  bin_pt=0  preci_type=Single  exp_width=8  frac_width=24  explicit_period=on  period=1  XmcBlockStatus=1  maskContainerNames=tabcontainer1  block_type=constant  block_config=sysgen:Constant_config
  Constant5 : hdlBasic/Constant  const=1  gui_display_data_type=Fixed-point  arith_type=Unsigned  n_bits=2  bin_pt=0  preci_type=Single  exp_width=8  frac_width=24  explicit_period=on  period=1  XmcBlockStatus=1  maskContainerNames=tabcontainer1  block_type=constant  block_config=sysgen:Constant_config
  Constant6 : hdlBasic/Constant  const=2  gui_display_data_type=Fixed-point  arith_type=Unsigned  n_bits=2  bin_pt=0  preci_type=Single  exp_width=8  frac_width=24  explicit_period=on  period=1  XmcBlockStatus=1  maskContainerNames=tabcontainer1  block_type=constant  block_config=sysgen:Constant_config
  Constant7 : hdlBasic/Constant  const=3  gui_display_data_type=Fixed-point  arith_type=Unsigned  n_bits=2  bin_pt=0  preci_type=Single  exp_width=8  frac_width=24  explicit_period=on  period=1  XmcBlockStatus=1  maskContainerNames=tabcontainer1  block_type=constant  block_config=sysgen:Constant_config
  Delay : hdlBasic/Delay  rst=off  en=off  latency=2  reg_retiming=off  XmcBlockStatus=1  maskContainerNames=group1  block_type=delay  block_config=sysgen:Delay_config
  Delay1 : hdlBasic/Delay  rst=off  en=off  latency=2  reg_retiming=off  XmcBlockStatus=1  maskContainerNames=group1  block_type=delay  block_config=sysgen:Delay_config
  Dual Port RAM{,1..3} (4 alike) : hdlBasic/Dual Port RAM  depth=16  initVector=zeros(1, 16)  distributed_mem=Block RAM  init_a=0  init_b=0  rst_a=off  rst_b=off  en_a=off  en_b=off  latency=1  write_mode_A=Read After Write  write_mode_B=Read After Write  explicit_period=[]  period=[]  simulation_type=fast_sim  XmcBlockStatus=1  maskContainerNames=tabcontainer1  block_type=dpram  block_config=sysgen:Dpram_config  optimize=Area
      settings: infoedit=[]
  Logical{,1..3} (4 alike) : hdlBasic/Logical  logical_function=AND  inputs=2  en=off  latency=1  precision=Full  arith_type=Unsigned  n_bits=16  bin_pt=0  align_bp=on  overflow=[]  quantization=[]  XmcBlockStatus=1  maskContainerNames=tabcontainer1  block_type=logical  block_config=sysgen:Logical_config
  Relational{,1..3} (4 alike) : hdlBasic/Relational  mode=a=b  op_type=Bool  en=off  latency=1  XmcBlockStatus=1  maskContainerNames=tabcontainer1  block_type=relational  block_config=sysgen:Relational_config
  Scalar to Vector{,1..3} (4 alike) : hdlSSR/Scalar2Vector  Width=18  sg_ssr=16  block_type=scalar2vector_ssr  XmcBlockStatus=1  sg_ssr_prev=16  maskContainerNames=group1
  Slice : hdlBasic/Slice  nbits=2  boolean_output=off  mode=Upper Bit Location + Width  bit1=0  base1=MSB of Input  bit0=0  base0=LSB of Input  XmcBlockStatus=1  maskContainerNames=group1  block_type=slice  block_config=sysgen:Slice_config
  Slice1 : hdlBasic/Slice  nbits=4  boolean_output=off  mode=Upper Bit Location + Width  bit1=-2  base1=MSB of Input  bit0=0  base0=LSB of Input  XmcBlockStatus=1  maskContainerNames=group1  block_type=slice  block_config=sysgen:Slice_config
  Terminator{,1..3} (4 alike) : Terminator
  Vector Reinterpret : hdlSSR/Vector Reinterpret  force_arith_type=on  arith_type=Unsigned  force_bin_pt=on  bin_pt=0  sg_ssr=16  block_type=reinterpret_ssr  XmcBlockStatus=1  sg_ssr_prev=16  maskContainerNames=group1
  Vector Reinterpret{1..4} (4 alike) : hdlSSR/Vector Reinterpret  force_arith_type=on  arith_type="Signed  (2's comp)"  force_bin_pt=on  bin_pt=17  sg_ssr=16  block_type=reinterpret_ssr  XmcBlockStatus=1  sg_ssr_prev=16  maskContainerNames=group1
  Vector to Scalar : hdlSSR/Vector2Scalar  sg_ssr=16  block_type=vector2scalar_ssr  XmcBlockStatus=1  sg_ssr_prev=16  maskContainerNames=group1
  d_out_a : Outport
  d_out_b : Outport  Port=2
  d_out_c : Outport  Port=3
  d_out_d : Outport  Port=4
  wires:
  addr_r_b/1 -> Dual Port RAM1/4
  Constant12/1 -> Dual Port RAM3/5
  addr_r_c/1 -> Dual Port RAM2/4
  Relational/1 -> Logical/2
  Constant6/1 -> Relational2/2
  Dual Port RAM1/1 -> Terminator1/1
  Constant11/1 -> Dual Port RAM2/5
  Vector Reinterpret/1 -> Vector to Scalar/1
  Relational3/1 -> Logical3/2
  Constant7/1 -> Relational3/2
  Dual Port RAM/1 -> Terminator/1
  Delay/1 -> Dual Port RAM3/1, Dual Port RAM2/1, Dual Port RAM1/1, Dual Port RAM/1
  Vector to Scalar/1 -> Delay1/1
  Logical2/1 -> Dual Port RAM2/3
  d_in/1 -> Vector Reinterpret/1
  Constant3/1 -> Dual Port RAM2/6
  Dual Port RAM1/2 -> Scalar to Vector1/1
  Delay1/1 -> Dual Port RAM3/2, Dual Port RAM2/2, Dual Port RAM1/2, Dual Port RAM/2
  Relational1/1 -> Logical1/2
  we/1 -> Logical3/1, Logical2/1, Logical1/1, Logical/1
  Slice/1 -> Relational3/1, Relational2/1, Relational1/1, Relational/1
  Constant9/1 -> Dual Port RAM/5
  Constant1/1 -> Dual Port RAM/6
  Dual Port RAM2/1 -> Terminator2/1
  Constant10/1 -> Dual Port RAM1/5
  w_addr/1 -> Slice1/1, Slice/1
  Dual Port RAM3/2 -> Scalar to Vector3/1
  Logical/1 -> Dual Port RAM/3
  Constant2/1 -> Dual Port RAM1/6
  Constant8/1 -> Dual Port RAM3/6
  Constant4/1 -> Relational/2
  Dual Port RAM3/1 -> Terminator3/1
  Logical1/1 -> Dual Port RAM1/3
  Logical3/1 -> Dual Port RAM3/3
  Constant5/1 -> Relational1/2
  Dual Port RAM2/2 -> Scalar to Vector2/1
  addr_r_d/1 -> Dual Port RAM3/4
  Slice1/1 -> Delay/1
  Relational2/1 -> Logical2/2
  addr_r_a/1 -> Dual Port RAM/4
  Dual Port RAM/2 -> Scalar to Vector/1
  Scalar to Vector/1 -> Vector Reinterpret1/1
  Scalar to Vector1/1 -> Vector Reinterpret2/1
  Scalar to Vector2/1 -> Vector Reinterpret3/1
  Scalar to Vector3/1 -> Vector Reinterpret4/1
  Vector Reinterpret1/1 -> d_out_a/1
  Vector Reinterpret2/1 -> d_out_b/1
  Vector Reinterpret3/1 -> d_out_c/1
  Vector Reinterpret4/1 -> d_out_d/1

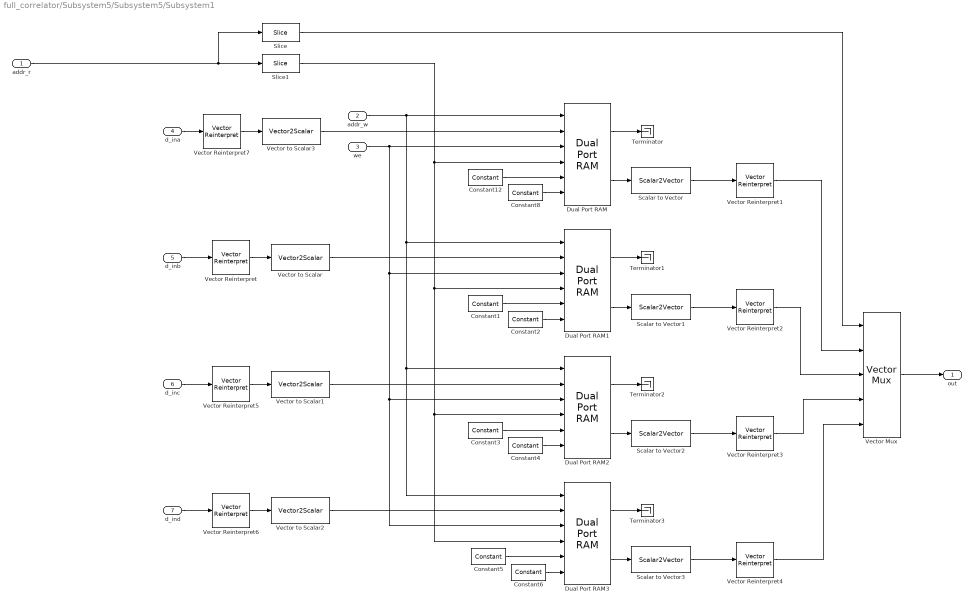
== system full_correlator/Subsystem5/Subsystem5/Subsystem1 ==
  addr_r : Inport
  addr_w : Inport  Port=2
  we : Inport  Port=3
  d_ina : Inport  Port=4
  d_inb : Inport  Port=5
  d_inc : Inport  Port=6
  d_ind : Inport  Port=7
  Constant{1,3,5,12} (4 alike) : hdlBasic/Constant  const=0  gui_display_data_type=Fixed-point  arith_type=Unsigned  n_bits=288  bin_pt=0  preci_type=Single  exp_width=8  frac_width=24  explicit_period=on  period=1  XmcBlockStatus=1  maskContainerNames=tabcontainer1  block_type=constant  block_config=sysgen:Constant_config
  Constant{2,4,6,8} (4 alike) : hdlBasic/Constant  const=0  gui_display_data_type=Boolean  arith_type=Boolean  n_bits=16  bin_pt=14  preci_type=Single  exp_width=8  frac_width=24  explicit_period=on  period=1  XmcBlockStatus=1  maskContainerNames=tabcontainer1  block_type=constant  block_config=sysgen:Constant_config
  Dual Port RAM{,1..3} (4 alike) : hdlBasic/Dual Port RAM  depth=16  initVector=zeros(1, 16)  distributed_mem=Block RAM  init_a=0  init_b=0  rst_a=off  rst_b=off  en_a=off  en_b=off  latency=1  write_mode_A=Read After Write  write_mode_B=Read After Write  explicit_period=[]  period=[]  simulation_type=fast_sim  XmcBlockStatus=1  maskContainerNames=tabcontainer1  block_type=dpram  block_config=sysgen:Dpram_config  optimize=Area
      settings: infoedit=[]
  Scalar to Vector{,1..3} (4 alike) : hdlSSR/Scalar2Vector  Width=18  sg_ssr=16  block_type=scalar2vector_ssr  XmcBlockStatus=1  sg_ssr_prev=16  maskContainerNames=group1
  Slice : hdlBasic/Slice  nbits=2  boolean_output=off  mode=Upper Bit Location + Width  bit1=0  base1=MSB of Input  bit0=0  base0=LSB of Input  XmcBlockStatus=1  maskContainerNames=group1  block_type=slice  block_config=sysgen:Slice_config
  Slice1 : hdlBasic/Slice  nbits=4  boolean_output=off  mode=Upper Bit Location + Width  bit1=-2  base1=MSB of Input  bit0=0  base0=LSB of Input  XmcBlockStatus=1  maskContainerNames=group1  block_type=slice  block_config=sysgen:Slice_config
  Terminator{,1..3} (4 alike) : Terminator
  Vector Mux : hdlSSR/Vector Mux  inputs=4  en=off  vectorize_en=off  vectorize_sel=off  sg_latency=1  sg_ssr=16  precision=Full  arith_type=Unsigned  n_bits=16  bin_pt=14  quantization=Truncate  overflow=Wrap  block_type=mux_ssr  inputs_prev=2  XmcBlockStatus=1  sg_ssr_prev=16  maskContainerNames=group1
  Vector Reinterpret{,5..7} (4 alike) : hdlSSR/Vector Reinterpret  force_arith_type=on  arith_type=Unsigned  force_bin_pt=on  bin_pt=0  sg_ssr=16  block_type=reinterpret_ssr  XmcBlockStatus=1  sg_ssr_prev=16  maskContainerNames=group1
  Vector Reinterpret{1..4} (4 alike) : hdlSSR/Vector Reinterpret  force_arith_type=on  arith_type="Signed  (2's comp)"  force_bin_pt=on  bin_pt=17  sg_ssr=16  block_type=reinterpret_ssr  XmcBlockStatus=1  sg_ssr_prev=16  maskContainerNames=group1
  Vector to Scalar{,1..3} (4 alike) : hdlSSR/Vector2Scalar  sg_ssr=16  block_type=vector2scalar_ssr  XmcBlockStatus=1  sg_ssr_prev=16  maskContainerNames=group1
  out : Outport
  wires:
  Dual Port RAM1/1 -> Terminator1/1
  Dual Port RAM/1 -> Terminator/1
  Dual Port RAM1/2 -> Scalar to Vector1/1
  Dual Port RAM2/1 -> Terminator2/1
  Dual Port RAM3/2 -> Scalar to Vector3/1
  Dual Port RAM3/1 -> Terminator3/1
  Dual Port RAM2/2 -> Scalar to Vector2/1
  Dual Port RAM/2 -> Scalar to Vector/1
  Scalar to Vector/1 -> Vector Reinterpret1/1
  Scalar to Vector1/1 -> Vector Reinterpret2/1
  Scalar to Vector2/1 -> Vector Reinterpret3/1
  Scalar to Vector3/1 -> Vector Reinterpret4/1
  addr_w/1 -> Dual Port RAM3/1, Dual Port RAM2/1, Dual Port RAM1/1, Dual Port RAM/1
  Vector to Scalar3/1 -> Dual Port RAM/2
  Vector to Scalar/1 -> Dual Port RAM1/2
  Vector to Scalar1/1 -> Dual Port RAM2/2
  Vector to Scalar2/1 -> Dual Port RAM3/2
  we/1 -> Dual Port RAM3/3, Dual Port RAM2/3, Dual Port RAM1/3, Dual Port RAM/3
  Vector Reinterpret/1 -> Vector to Scalar/1
  Vector Reinterpret5/1 -> Vector to Scalar1/1
  Vector Reinterpret6/1 -> Vector to Scalar2/1
  Vector Reinterpret7/1 -> Vector to Scalar3/1
  Vector Mux/1 -> out/1
  Vector Reinterpret1/1 -> Vector Mux/2
  Vector Reinterpret2/1 -> Vector Mux/3
  Vector Reinterpret3/1 -> Vector Mux/4
  Vector Reinterpret4/1 -> Vector Mux/5
  Constant8/1 -> Dual Port RAM/6
  Constant12/1 -> Dual Port RAM/5
  Constant2/1 -> Dual Port RAM1/6
  Constant1/1 -> Dual Port RAM1/5
  Constant4/1 -> Dual Port RAM2/6
  Constant3/1 -> Dual Port RAM2/5
  Constant6/1 -> Dual Port RAM3/6
  Constant5/1 -> Dual Port RAM3/5
  addr_r/1 -> Slice/1, Slice1/1
  Slice/1 -> Vector Mux/1
  Slice1/1 -> Dual Port RAM3/4, Dual Port RAM2/4, Dual Port RAM1/4, Dual Port RAM/4
  d_ina/1 -> Vector Reinterpret7/1
  d_inb/1 -> Vector Reinterpret/1
  d_inc/1 -> Vector Reinterpret5/1
  d_ind/1 -> Vector Reinterpret6/1

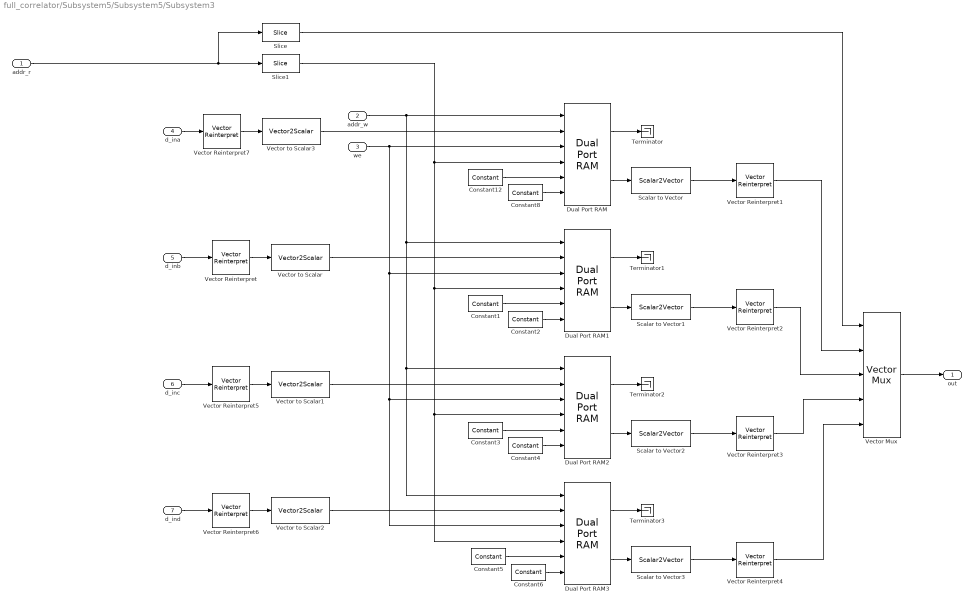
== system full_correlator/Subsystem5/Subsystem5/Subsystem3 ==
  addr_r : Inport
  addr_w : Inport  Port=2
  we : Inport  Port=3
  d_ina : Inport  Port=4
  d_inb : Inport  Port=5
  d_inc : Inport  Port=6
  d_ind : Inport  Port=7
  Constant{1,3,5,12} (4 alike) : hdlBasic/Constant  const=0  gui_display_data_type=Fixed-point  arith_type=Unsigned  n_bits=288  bin_pt=0  preci_type=Single  exp_width=8  frac_width=24  explicit_period=on  period=1  XmcBlockStatus=1  maskContainerNames=tabcontainer1  block_type=constant  block_config=sysgen:Constant_config
  Constant{2,4,6,8} (4 alike) : hdlBasic/Constant  const=0  gui_display_data_type=Boolean  arith_type=Boolean  n_bits=16  bin_pt=14  preci_type=Single  exp_width=8  frac_width=24  explicit_period=on  period=1  XmcBlockStatus=1  maskContainerNames=tabcontainer1  block_type=constant  block_config=sysgen:Constant_config
  Dual Port RAM{,1..3} (4 alike) : hdlBasic/Dual Port RAM  depth=16  initVector=zeros(1, 16)  distributed_mem=Block RAM  init_a=0  init_b=0  rst_a=off  rst_b=off  en_a=off  en_b=off  latency=1  write_mode_A=Read After Write  write_mode_B=Read After Write  explicit_period=[]  period=[]  simulation_type=fast_sim  XmcBlockStatus=1  maskContainerNames=tabcontainer1  block_type=dpram  block_config=sysgen:Dpram_config  optimize=Area
      settings: infoedit=[]
  Scalar to Vector{,1..3} (4 alike) : hdlSSR/Scalar2Vector  Width=18  sg_ssr=16  block_type=scalar2vector_ssr  XmcBlockStatus=1  sg_ssr_prev=16  maskContainerNames=group1
  Slice : hdlBasic/Slice  nbits=2  boolean_output=off  mode=Upper Bit Location + Width  bit1=0  base1=MSB of Input  bit0=0  base0=LSB of Input  XmcBlockStatus=1  maskContainerNames=group1  block_type=slice  block_config=sysgen:Slice_config
  Slice1 : hdlBasic/Slice  nbits=4  boolean_output=off  mode=Upper Bit Location + Width  bit1=-2  base1=MSB of Input  bit0=0  base0=LSB of Input  XmcBlockStatus=1  maskContainerNames=group1  block_type=slice  block_config=sysgen:Slice_config
  Terminator{,1..3} (4 alike) : Terminator
  Vector Mux : hdlSSR/Vector Mux  inputs=4  en=off  vectorize_en=off  vectorize_sel=off  sg_latency=1  sg_ssr=16  precision=Full  arith_type=Unsigned  n_bits=16  bin_pt=14  quantization=Truncate  overflow=Wrap  block_type=mux_ssr  inputs_prev=2  XmcBlockStatus=1  sg_ssr_prev=16  maskContainerNames=group1
  Vector Reinterpret{,5..7} (4 alike) : hdlSSR/Vector Reinterpret  force_arith_type=on  arith_type=Unsigned  force_bin_pt=on  bin_pt=0  sg_ssr=16  block_type=reinterpret_ssr  XmcBlockStatus=1  sg_ssr_prev=16  maskContainerNames=group1
  Vector Reinterpret{1..4} (4 alike) : hdlSSR/Vector Reinterpret  force_arith_type=on  arith_type="Signed  (2's comp)"  force_bin_pt=on  bin_pt=17  sg_ssr=16  block_type=reinterpret_ssr  XmcBlockStatus=1  sg_ssr_prev=16  maskContainerNames=group1
  Vector to Scalar{,1..3} (4 alike) : hdlSSR/Vector2Scalar  sg_ssr=16  block_type=vector2scalar_ssr  XmcBlockStatus=1  sg_ssr_prev=16  maskContainerNames=group1
  out : Outport
  wires:
  Dual Port RAM1/1 -> Terminator1/1
  Dual Port RAM/1 -> Terminator/1
  Dual Port RAM1/2 -> Scalar to Vector1/1
  Dual Port RAM2/1 -> Terminator2/1
  Dual Port RAM3/2 -> Scalar to Vector3/1
  Dual Port RAM3/1 -> Terminator3/1
  Dual Port RAM2/2 -> Scalar to Vector2/1
  Dual Port RAM/2 -> Scalar to Vector/1
  Scalar to Vector/1 -> Vector Reinterpret1/1
  Scalar to Vector1/1 -> Vector Reinterpret2/1
  Scalar to Vector2/1 -> Vector Reinterpret3/1
  Scalar to Vector3/1 -> Vector Reinterpret4/1
  addr_w/1 -> Dual Port RAM3/1, Dual Port RAM2/1, Dual Port RAM1/1, Dual Port RAM/1
  Vector to Scalar3/1 -> Dual Port RAM/2
  Vector to Scalar/1 -> Dual Port RAM1/2
  Vector to Scalar1/1 -> Dual Port RAM2/2
  Vector to Scalar2/1 -> Dual Port RAM3/2
  we/1 -> Dual Port RAM3/3, Dual Port RAM2/3, Dual Port RAM1/3, Dual Port RAM/3
  Vector Reinterpret/1 -> Vector to Scalar/1
  Vector Reinterpret5/1 -> Vector to Scalar1/1
  Vector Reinterpret6/1 -> Vector to Scalar2/1
  Vector Reinterpret7/1 -> Vector to Scalar3/1
  Vector Mux/1 -> out/1
  Vector Reinterpret1/1 -> Vector Mux/2
  Vector Reinterpret2/1 -> Vector Mux/3
  Vector Reinterpret3/1 -> Vector Mux/4
  Vector Reinterpret4/1 -> Vector Mux/5
  Constant8/1 -> Dual Port RAM/6
  Constant12/1 -> Dual Port RAM/5
  Constant2/1 -> Dual Port RAM1/6
  Constant1/1 -> Dual Port RAM1/5
  Constant4/1 -> Dual Port RAM2/6
  Constant3/1 -> Dual Port RAM2/5
  Constant6/1 -> Dual Port RAM3/6
  Constant5/1 -> Dual Port RAM3/5
  addr_r/1 -> Slice/1, Slice1/1
  Slice/1 -> Vector Mux/1
  Slice1/1 -> Dual Port RAM3/4, Dual Port RAM2/4, Dual Port RAM1/4, Dual Port RAM/4
  d_ina/1 -> Vector Reinterpret7/1
  d_inb/1 -> Vector Reinterpret/1
  d_inc/1 -> Vector Reinterpret5/1
  d_ind/1 -> Vector Reinterpret6/1
